simulink model "Understanding_and_playing"  (R2022b)
settings: Solver=VariableStepAuto  StartTime=0.0  StopTime=15  RelTol=1e-3
model workspace (MAT data in the model file):
  Inertia = [0.001  0  0; 0  0.001  0; 0  0  0.001]
  M = 1
  R_CoM = [1; 1; 0]
  Td = Simulink.Parameter
  Td.Value = 0.01
  Td.DataType = 'double'
  Td.Complexity = 'real'
  Td.Dimensions = [1 1]
  g = [0; 0; -9.81]
libraries: simulink x4, vrlib x3, sharedtransform x2, dspindex x2, shared6dof x1, matrix_library x1, aerolibanim x1
settings Model: PacingRate=0.500000  Creator=david  LastModifiedBy=david

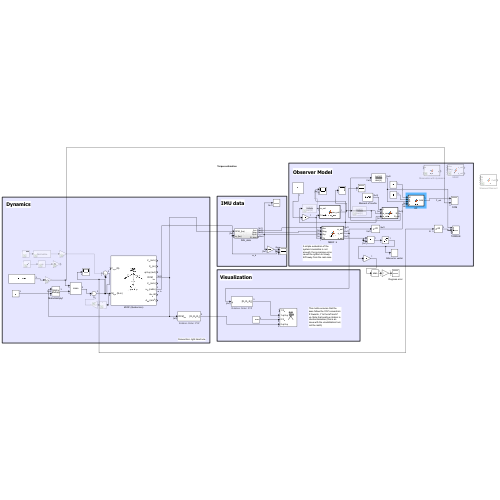
[thumbnail: Simulink's stored preview of the top-level diagram]
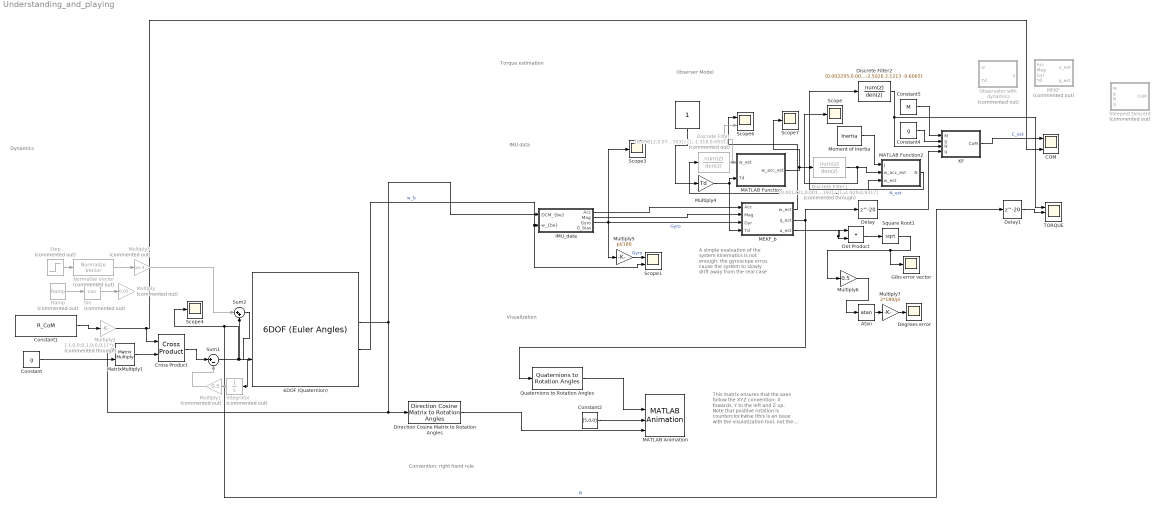
== system Understanding_and_playing ==
  note: Torque estimation
  note: Convention: right hand rule
  note: A simple evaluation of the system kinematics is not enough: the gyroscope erros cause the system to slowly drift away from the real case
  note: Dynamics
  note: This matrix ensures that the axes follow the XYZ convention: X fowards, Y to the left and Z up. Note that positive rotation is counterclockwise (this is an issue with the visulatization tool, not the math)
  note: Observer Model
  note: Visualization
  note: IMU data
  " " : Constant
  6DOF (Quaternion) : shared6dof/6DOF (Euler Angles)  units=Metric (MKS)  mtype=Fixed  rep=Quaternion  xme_0=[0 0 0]  Vm_0=[0 0 0]  eul_0=[0 0 0]  pm_0=[0 0 0]  mass_0=M  mass_e=0.5  mass_f=2.0  inertia=Inertia  inertia_e=eye(3)  inertia_f=2*eye(3)  k_quat=1.0  vre_flag=on  abi_flag=off  aMode=0  xme_statename=''  Vm_statename=''  eul_statename=''  quat_statename=''  pm_statename=''  mass_statename=''
      settings: LibrarySourceBlock=aerolib6dof2/6DOF (Quaternion)
  Atan : Trigonometry  Operator=atan
  COM : Scope  NumInputPorts=2
  Constant : Constant  Value=g
  Constant1 : Constant  Value=R_CoM
  Constant2 : Constant  Value=[5,0,0]
  Constant4 : Constant  Value=g
  Constant5 : Constant  Value=M
  Cross Product : matrix_library/Cross Product
  Degrees error : Scope
  Delay : Delay  DelayLength=20
  Delay1 : Delay  DelayLength=20
  Direction Cosine Matrix to Rotation Angles : sharedtransform/Direction Cosine Matrix to Rotation Angles  rotationOrder=XYZ  aMode=aMode  action=None  tolerance=eps(2)
      settings: LibrarySourceBlock=|
      | aerolibtransform2/Direction Cosine Matrix
      | to Rotation Angles
  Discrete Filter : DiscreteFilter  Commented=on  Numerator=[0.09812,0.07743]  Denominator=[1,-1.318,0.4931]
  Discrete Filter1 : DiscreteFilter  Commented=through  Numerator=[0.001221,0.001192]  Denominator=[1,-1.929,0.9317]
  Discrete Filter2 : DiscreteFilter  Numerator=[0.002295,0.008087,0.001787]  Denominator=[1 -2.5026 2.1213 -0.6065]
  Dot Product : DotProduct  OutDataTypeStr=Inherit: Inherit via internal rule
  Gibs error vector : Scope
  IMU_data : Subsystem
  Integrator : Integrator  Commented=on
  KF : MATLAB Function  TreatAsAtomicUnit=on
  MATLAB Animation : aerolibanim/MATLAB Animation  Tag=Matlab Animation 6 DOF  Vehicles=2  Geometries={'astredwedge.mat','astredwedge.mat'}  BoundingBoxCoordinates=[-50,50,-50,50,-50,50]  CameraOffset=[150,150,0]  CameraViewAngle=3  SampleTime=0.01  FigurePosition=[765,4.180000e+01,7.664000e+02,7.664000e+02]
  MATLAB Function : MATLAB Function  TreatAsAtomicUnit=on
  MATLAB Function2 : MATLAB Function  TreatAsAtomicUnit=on
  MEKF : MATLAB Function  Commented=on  TreatAsAtomicUnit=on  SystemSampleTime=Td
  MEKF_b : MATLAB Function  TreatAsAtomicUnit=on  SystemSampleTime=Td
  MatrixMultiply1 : Product  Multiplication=Matrix(*)
  Moment of Inertia : Constant  Value=Inertia
  Multiply : Gain  Commented=on  Gain=0.05
  Multiply1 : Gain  Commented=on  Gain=0.5
  Multiply2 : Gain  Commented=through  Gain=[-1,0,0;0,1,0;0,0,1]  Multiplication=Matrix(K*u)
  Multiply3 : Gain  Commented=on  Gain=1e-3
  Multiply4 : Gain  Gain=Td
  Multiply5 : Gain  Gain=pi/180
  Multiply6 : Gain  Gain=0.5
  Multiply7 : Gain  Gain=2*180/pi
  Normalize Vector : vrlib/Utilities/Normalize Vector  Commented=on  maxzero=0
  Observator with dynamics : MATLAB Function  Commented=on  TreatAsAtomicUnit=on  SystemSampleTime=Td
  Quaternions to Rotation Angles : sharedtransform/Quaternions to Rotation Angles  rotationOrder=XYZ  aMode=aMode
  Ramp : simulink/Sources/Ramp  Commented=on  slope=[1,0,0]*2*pi/30  start=0  InitialOutput=[0,pi/2,pi/2]
  Scope{,3..4,7} (4 alike) : Scope
  Scope1 : Scope  NumInputPorts=2
  Scope6 : Scope  NumInputPorts=2
  Sin : Trigonometry  Commented=on  Operator=cos
  Square Root1 : Sqrt
  Steepest Descent : MATLAB Function  Commented=on  TreatAsAtomicUnit=on
  Step : Step  Commented=on  Before=[0,0,1]  After=[0,0,0]  SampleTime=0
  Sum1 : Sum  Inputs=|+-
  Sum2 : Sum  Inputs=|++
  TORQUE : Scope  NumInputPorts=3
  wires:
  6DOF (Quaternion)/4 -> MatrixMultiply1/1, Direction Cosine Matrix to Rotation Angles/1, IMU_data/1("DCM_{be}")
  Step/1 -> Normalize Vector/1
  Direction Cosine Matrix to Rotation Angles/1 -> MATLAB Animation/4
  Constant2/1 -> MATLAB Animation/3
  6DOF (Quaternion)/6 -> Scope1/2, IMU_data/2("w_{be}")  "w_b"
  Quaternions to Rotation Angles/1 -> MATLAB Animation/2
  " "/1 -> Multiply4/1
  IMU_data/3(Gyro) -> Scope3/1, MEKF_b/3(Gyr), Multiply5/1  "Gyro"
  Multiply4/1 -> MEKF_b/4(Td), MATLAB Function/2(Td)
  Multiply5/1 -> Scope1/1  "Gyro"
  IMU_data/1(Acc) -> MEKF_b/1(Acc)
  IMU_data/2(Mag) -> MEKF_b/2(Mag)
  MEKF_b/3(a_est) -> Dot Product/2, Dot Product/1
  Dot Product/1 -> Square Root1/1
  MATLAB Function/1(w_acc_est) -> Scope7/1, Discrete Filter1/1
  Discrete Filter1/1 -> MATLAB Function2/2(w_acc_est), Scope/1
  Moment of Inertia/1 -> MATLAB Function2/1(J)
  MEKF_b/1(w_est) -> Scope6/1, MATLAB Function2/3(w_est), Discrete Filter/1
  MATLAB Function2/1(N) -> Discrete Filter2/1  "N_est"
  Discrete Filter/1 -> Scope6/2, MATLAB Function/1(w_est)
  Square Root1/1 -> Multiply6/1, Gibs error vector/1
  Sin/1 -> Multiply/1
  Ramp/1 -> Sin/1
  Constant/1 -> MatrixMultiply1/2
  MatrixMultiply1/1 -> Cross Product/2
  Constant1/1 -> Multiply2/1
  Cross Product/1 -> Sum1/1
  Sum1/1 -> Delay1/1, Scope4/1, Integrator/1, Sum2/2  "N"
  Integrator/1 -> Multiply1/1
  Multiply1/1 -> Sum1/2
  Multiply2/1 -> COM/2, Cross Product/1
  KF/1(CoM) -> COM/1  "C_est"
  Constant4/1 -> KF/2(g)
  Normalize Vector/1 -> Multiply3/1
  Sum2/1 -> 6DOF (Quaternion)/2
  Multiply3/1 -> Sum2/1
  Constant5/1 -> KF/1(M)
  Discrete Filter2/1 -> KF/3(N), TORQUE/1
  MEKF_b/2(q_est) -> Delay/1, Quaternions to Rotation Angles/1
  Delay/1 -> KF/4(q)
  Delay1/1 -> TORQUE/2
  Multiply6/1 -> Atan/1
  Atan/1 -> Multiply7/1
  Multiply7/1 -> Degrees error/1

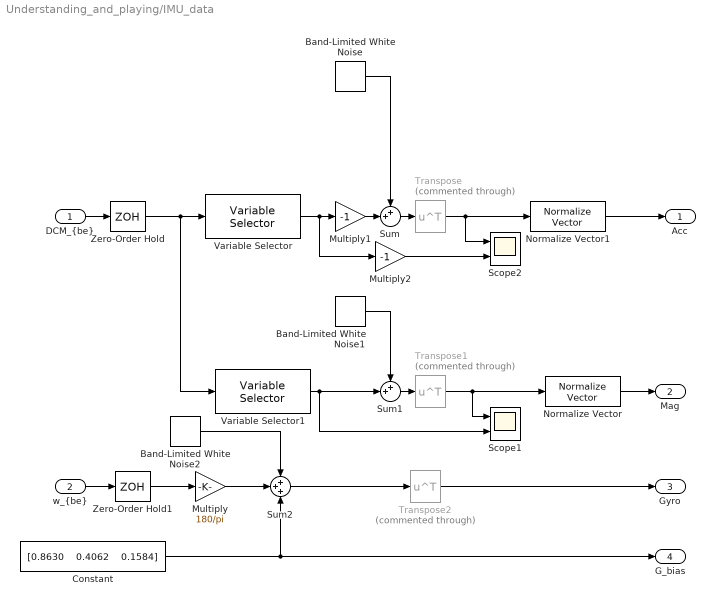
== system Understanding_and_playing/IMU_data ==
  "DCM_{be}" : Inport
  "w_{be}" : Inport  Port=2
  Band-Limited White Noise : simulink/Sources/Band-Limited White Noise  Cov="[0.0515  ;  0.0423  ;  0.1177]*1e-4"  Ts=Td  seed=[23341;23342;23343]  VectorParams1D=off
  Band-Limited White Noise1 : simulink/Sources/Band-Limited White Noise  Cov="[0.2967  ;  0.1789 ;   0.2126]*1e-4"  Ts=Td  seed=[23344;23345;26343]  VectorParams1D=off
  Band-Limited White Noise2 : simulink/Sources/Band-Limited White Noise  Cov="[0.0149;    0.0162;    0.0127]"  Ts=Td  seed=[21341;22342;33343]  VectorParams1D=off
  Constant : Constant  Value="[0.8630    0.4062    0.1584]"  SampleTime=Td
  Multiply : Gain  Gain=180/pi
  Multiply1 : Gain  Gain=-1
  Multiply2 : Gain  Gain=-1
  Normalize Vector : vrlib/Utilities/Normalize Vector  maxzero=0
  Normalize Vector1 : vrlib/Utilities/Normalize Vector  maxzero=0
  Scope1 : Scope  NumInputPorts=2
  Scope2 : Scope  NumInputPorts=2
  Sum : Sum  Inputs=++|
  Sum1 : Sum  Inputs=++|
  Sum2 : Sum  Inputs=+++
  Transpose : Math  Commented=through  Operator=transpose
  Transpose1 : Math  Commented=through  Operator=transpose
  Transpose2 : Math  Commented=through  Operator=transpose
  Variable Selector : dspindex/Variable Selector  NumInputs=1  rowsOrCols=Columns  IdxMode=Fixed  Elements=[3]  ZerOneIdxMode=One-based  errmode=Clip Index  FillMode=on  FillValues=0
  Variable Selector1 : dspindex/Variable Selector  NumInputs=1  rowsOrCols=Columns  IdxMode=Fixed  Elements=[1]  ZerOneIdxMode=One-based  errmode=Clip Index  FillMode=on  FillValues=0
  Zero-Order Hold : ZeroOrderHold  SampleTime=Td
  Zero-Order Hold1 : ZeroOrderHold  SampleTime=Td
  Acc : Outport
  Mag : Outport  Port=2
  Gyro : Outport  Port=3
  G_bias : Outport  Port=4
  wires:
  Variable Selector/1 -> Multiply2/1, Multiply1/1
  Multiply2/1 -> Scope2/2
  Multiply1/1 -> Sum/2
  "DCM_{be}"/1 -> Zero-Order Hold/1
  Zero-Order Hold/1 -> Variable Selector1/1, Variable Selector/1
  Band-Limited White Noise1/1 -> Sum1/1
  Variable Selector1/1 -> Sum1/2, Scope1/2
  "w_{be}"/1 -> Zero-Order Hold1/1
  Band-Limited White Noise2/1 -> Sum2/1
  Sum2/1 -> Transpose2/1
  Sum/1 -> Transpose/1
  Sum1/1 -> Transpose1/1
  Transpose2/1 -> Gyro/1
  Band-Limited White Noise/1 -> Sum/1
  Constant/1 -> G_bias/1, Sum2/3
  Normalize Vector1/1 -> Acc/1
  Multiply/1 -> Sum2/2
  Zero-Order Hold1/1 -> Multiply/1
  Normalize Vector/1 -> Mag/1
  Transpose/1 -> Normalize Vector1/1, Scope2/1
  Transpose1/1 -> Normalize Vector/1, Scope1/1

== matlab function Understanding_and_playing/Observator with dynamics ==
  settings: updateMethod=DISCRETE  sampleTime=Td
  data: w input; q output; Td input
function q = fcn(w,Td)
% Input q0 follows [q(1:3),q(4)] as a column vector (our way)
% Input w is a column vector of BODY rotation speed
%Output q follows [q(4),q(1:3)] as a column vector (Matlab way)
    persistent q_state

    if isempty(q_state)
    q_state = [0,0,0,1]';
    end
    q_state = (eye(4,4)+Td/2*skew4([w;0]/180*pi))*q_state;
    q_state = q_state/norm(q_state);
    q = [q_state(4);q_state(1:3)];

== matlab function Understanding_and_playing/MEKF ==
  data: Acc input; Mag input; Gyr input; x_est output; Td input; q_est output
function [x_est,q_est] = fcn(Acc,Mag,Gyr,Td)
% Td is the time step
% Acc is the normalised vector of gravity.
% Mag is normalised, points to x coordinate
% Gyr  is in degrees/s, in body coordinates.
persistent q % q1,q2,q3,q4 with q4 as double
persistent x
persistent P
% Initialization
Q =diag([0.0149;    0.0162;    0.0127]/180*pi);
R = 0.01*eye(6);

if isempty(q)
    q = [0,0,0,1]';   % Initial Rotation
    q = q/norm(q);
end
if isempty(x)
    x = [0,0,0]'; % x = [a,b], with b as bias of gyro
end
if isempty(P)
    P = 2*eye(3,3);            % assume unkown initial state
end
% Correc units and direction: right hand rule
Gyr = Gyr/180*pi % º to rads/s
% Update state
q = (eye(4,4)+Td/2*skew4([Gyr;0]))*q; %Notice that this equation follows the left hand rule, so the minus is added
q = q/norm(q)
F = skew3(Gyr);
G = -eye(3,3);
P = P + Td*(F*P+P*F'+G*Q*G');

% Measurement state
A = (q(4)^2-norm(q(1:3))^2)*eye(3,3)+2*q(1:3)*q(1:3)'-2*q(4)*skew3(q(1:3));
Acc_est  = A*[0;0;-1]
Mag_est  = A*[1;0;0]
Ha = [skew3(Acc_est);skew3(Mag_est)];
H = Ha;

K = P*H'/(H*P*H'+R);
innovation = [Acc;Mag]-[Acc_est;Mag_est];
x = x + K*innovation;
P = P - K*H*P;
% Correction step
q_err = [x/2;1-norm(x)^2/8];
q = skew4(q_err)*q;
x_est = x;
x = zeros(3,1);

q_est = [q(4);q(1:3)];

== matlab function Understanding_and_playing/MEKF_b ==
  data: w_est output; Acc input; Mag input; Gyr input; Td input; q_est output; a_est output
function [w_est,q_est,a_est]  = MEKF(Acc,Mag,Gyr,Td)
% Td is the time step
% Acc is the normalised vector of gravity.
% Mag is normalised, points to x coordinate
% Gyr  is in degrees/s, in body coordinates.
persistent q % q1,q2,q3,q4 with q4 as double
persistent x
persistent P
% Initialization
%Q =diag([0.0149;    .0162;    0.0127; 0.01; 0.01; 0.01]/180*pi);
%R = 0.01*eye(6);
R = diag([0.0515  ;  0.0423  ;  0.1177; 0.2967  ;  0.1789 ;   0.2126]*1e-4);
Q = diag([0.0149;    0.0162;    0.0127;0.01;0.01;0.01]);
if isempty(q)
    q = [0,0,0.2,1]';   % Initial Rotation
    q = q/norm(q);
end
if isempty(x)
    x = [0,0,0,0,0,0]'; % x = [a,b], with b as bias of gyro
end
if isempty(P)
    P = diag([2,2,2,0,0,0]);            % assume unkown initial state
end

%if(norm(x(4:6))>4)
%    x(4:6) = x(4:6)/norm(x(4:6));
%end
% Corrected units
w_est = Gyr/180*pi-x(4:6); % º to rads/s
% Update state
q = (eye(4,4)+Td/2*skew4([w_est;0]))*q; %Notice that this equation follows the left hand rule, so the minus is added
q = q/norm(q);
F = [skew3(w_est),-eye(3,3);zeros(3,6)];
G = [-eye(3,3),zeros(3,3);zeros(3,3),eye(3,3)];
P = P + Td*(F*P+P*F'+G*Q*G');

% Measurement state
A = (q(4)^2-norm(q(1:3))^2)*eye(3,3)+2*q(1:3)*q(1:3)'-2*q(4)*skew3(q(1:3));
Acc_est  = A*[0;0;-1];
Mag_est  = A*[1;0;0];
Ha = [skew3(Acc_est);skew3(Mag_est)];
H = [Ha,zeros(6,3)];

K = P*H'/(H*P*H'+R);
innovation = [Acc;Mag]-[Acc_est;Mag_est];
x = x + K*innovation;
P = P - K*H*P;
% Correction step
q_err = [x(1:3)/2;1-norm(x(1:3))^2/8];
q = skew4(q_err)*q;
x(1:3) = zeros(3,1);
a_est = Ha\innovation;
q_est = [q(4);q(1:3)];

== matlab function Understanding_and_playing/MATLAB Function ==
  data: w_acc_est output; w_est input; Td input
function w_acc_est = estimate_acc(w_est,Td)
persistent w_prev
if isempty(w_prev)
    w_prev = w_est;
end
w_acc_est = 1/Td*(w_est-w_prev);
w_prev = w_est;

== matlab function Understanding_and_playing/MATLAB Function2 ==
  data: J input; N output; w_acc_est input; w_est input
function N = fcn(J,w_acc_est,w_est)
    N = J*w_acc_est - cross(w_est,J*w_est);
end

== matlab function Understanding_and_playing/Steepest Descent ==
  data: M input; g input; N input; CoM output; q input
function CoM  = CoM(M,g,N,q)
persistent R
mu = 0.00005;
if isempty(R)
    R = [0;0;0];
end
q = [q(2:4);q(1)];
A = (q(4)^2-norm(q(1:3))^2)*eye(3,3)+2*q(1:3)*q(1:3)'-2*q(4)*skew3(q(1:3));
g_b = A*g;

R = R + mu*cross(g_b,cross(g_b,R*M)+N);
CoM = -R;
end

== matlab function Understanding_and_playing/KF ==
  data: M input; g input; N input; CoM output; q input
function CoM  = CoM(M,g,N,q)
% States: R (CoM)
% Inputs: none
% Outputs: N
persistent x
persistent P
if isempty(x)
    x = [0;0;0];
end
if isempty(P)
    P = eye(3,3);
end
q = [q(2:4);q(1)];
A = (q(4)^2-norm(q(1:3))^2)*eye(3,3)+2*q(1:3)*q(1:3)'-2*q(4)*skew3(q(1:3));
A*g
skew_g = -skew3(A*g);

Q = 0.01*eye(3,3);
R = eye(3,3);
% Update equations
x = x; % No update
F = eye(3,3);
H = skew_g*M;
P = F*P*F'+Q;
% Measurements equations
K = P*H'*inv((H*P*H'+R));
K
innov = N - H*M*x;
innov
x = x + K*innov;
P = (eye(3,3)-K*H)*P;


CoM = x;
end
